simulink model "PositionControlNet"  (R2019b)
settings: Solver=ode3  StartTime=0.0  StopTime=100.0  FixedStep=Ts  RelTol=1e-3
values from neighbouring files (symbols this model uses):
  refx = 2.0    (= 2)    [RunPositionControl_b.m]    (also in RunPositionControl_d.m; RunPositionControl_e.m = 10 * rand - 5; RunPositionControl_i.m = 10 * rand - 5)
  refy = 2.0    (= 2)    [RunPositionControl_b.m]    (also in RunPositionControl_d.m; RunPositionControl_e.m = 10 * rand - 5; RunPositionControl_i.m = 10 * rand - 5)
undefined symbols (not defined in the file or in its folder): DiscIntNeverNeededParam
libraries: neural x56, simulink x1
(part 2 of 2)

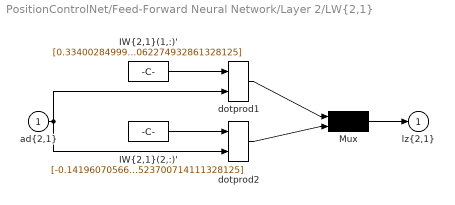
== system PositionControlNet/Feed-Forward Neural Network/Layer 2/LW{2,1} ==
  "ad{2,1}" : Inport  PortDimensions=50  SampleTime=0.1
      mask Display: e = 0.06;c1 = [120 230 180]/255;c2 = ([120 230 180]+0)/(256+128);c3 = ([120 230 180]+128)/(256+128);patch([0 1 1 0],[0 0 1 1],c1);patch([0 1 1 1-e 1-e 0+e],[0 0 1 1-e 0+e 0+e],c2);patch([0 0 1 1-e 0+e 0+e],[0 1 1 1-e 1-e 0+e],c3);plot([0 1 1 0 0],[0 0 1 1 0]);
  "IW{2,1}(1,:)'" : Constant  Value=[0.334002849994705253156013213811093010008335113525390625;-0.5040820987454741608502217786735855042934417724609375;-0.91935122834619387166554815848940052092075347900390625;0.32639735666295488503152455450617708265781402587890625;-0.187840693667216063200697817592299543321132659912109375;-0.11460469237998084646168450717595987953245639801025390625;0.717609320213467238858129348955117166042327880859375;1.3523732656893934223063524768804199993610382080078125;0.179703748271600349806220719983684830367565155029296875;-0.87500417966937893421430771923041902482509613037109375;-0.25199618840757465054736030651838518679141998291015625;-0.1195075191355988997177206556443707086145877838134765625;0.0728694591968338800658244736041524447500705718994140625;0.00809319958874362734013718778669499442912638187408447265625;-0.333437385428566102074654509124229662120342254638671875;0.0994025146375227264261553727919817902147769927978515625;-0.41078606437725884159561928754555992782115936279296875;0.60772390003159160176693376342882402241230010986328125;-0.50564194028696107796605474504758603870868682861328125;0.058621075153028744109118264304925105534493923187255859375;0.0248756429867585289461562325641352799721062183380126953125;-0.71916004594758631274231674979091621935367584228515625;-1.252886988501913823057520858128555119037628173828125;-0.1880074118303163566157110153653775341808795928955078125;0.1769309421471805532366516899855923838913440704345703125;0.47920092495693966672121177907683886587619781494140625;0.469176086459065333489348859075107611715793609619140625;0.377404235098586282592947327430010773241519927978515625;-0.406199561893793192890456111854291521012783050537109375;0.251041830696620227314497242332436144351959228515625;0.63316865040098979644511700826114974915981292724609375;-0.041829399940195056972758180791061022318899631500244140625;0.07987491955746865712750803822927991859614849090576171875;0.01011828325154251646822434196337781031616032123565673828125;0.0138200191255173875093387181323123513720929622650146484375;0.053368350017781542027339725109413848258554935455322265625;-0.62375837716052540127265046976390294730663299560546875;-0.045674105604766306043540424752791295759379863739013671875;-0.03509042242425212954071156445934320800006389617919921875;0.10806119620553211735369814050500281155109405517578125;-0.1630870104185702385013456705564749427139759063720703125;-0.11223416664183298585566461724738474003970623016357421875;-0.03950550369853102206096906456878059543669223785400390625;0.045018325314339573128830096493402379564940929412841796875;0.361073442667731503430417205890989862382411956787109375;-0.432799903513595152215742700718692503869533538818359375;0.984287018175489247795439951005391776561737060546875;0.125820475234998507829686786863021552562713623046875;-0.1203917071761672896723638359617325477302074432373046875;0.607004742466177305004748632200062274932861328125]
      mask Display: e = 0.06;c1 = [120 150 230]/255;c2 = ([120 150 230]+0)/383;c3 = ([120 150 230]+128)/383;patch([0 1 1 0],[0 0 1 1],c1);patch([0 1 1 1-e 1-e 0+e],[0 0 1 1-e 0+e 0+e],c2);patch([0 0 1 1-e 0+e 0+e],[0 1 1 1-e 1-e 0+e],c3);plot([0 1 1 0 0],[0 0 1 1 0]);disp('weights');
  "IW{2,1}(2,:)'" : Constant  Value=[-0.1419607056600145356117792516670306213200092315673828125;1.028827672248862068471453312668018043041229248046875;0.045383286118671088693599102725784177891910076141357421875;-0.218572716912245945675152825060649774968624114990234375;0.434083133810548360553838165287743322551250457763671875;0.50308140166235026935481755572254769504070281982421875;0.0201769956134996049368357518005723250098526477813720703125;0.04642214440832766186861846335887094028294086456298828125;-0.032438045155445953404704795275392825715243816375732421875;0.85025309020824313410713557459530420601367950439453125;-0.1201983909327605515304782102248282171785831451416015625;0.036994653062803813103887051738638547249138355255126953125;0.1300649198493276370580673528820625506341457366943359375;-0.344468723662421372200270752728101797401905059814453125;0.13513417310886577382689210935495793819427490234375;0.11122951518489221367502750581479631364345550537109375;-0.0789493036264423964087910690068383701145648956298828125;0.278793521052757231615260025137104094028472900390625;-0.08590393630611155295628833528098766691982746124267578125;0.0226878938136040701756268589406317914836108684539794921875;0.000776186346165941829823575748292796561145223677158355712890625;0.4489477159577852649618989744340069591999053955078125;0.1417734772799557896316713367923512123525142669677734375;-0.061852047013610460257648782089745509438216686248779296875;-0.2381090914265252267423278453861712478101253509521484375;0.274562097712392982895579507385264150798320770263671875;-0.0930798944562686025872011441606446169316768646240234375;-0.132101370043506471940730762071325443685054779052734375;0.0996268771357249616205109532529604621231555938720703125;0.261387848508712716810720166904502548277378082275390625;-0.0244297733572668984702858097080024890601634979248046875;-0.023142883803481929805290207013968029059469699859619140625;-0.0499752192089107649675128186572692357003688812255859375;-0.0179734345381963069032682511760867782868444919586181640625;0.014274641402173791904228750127003877423703670501708984375;0.129618086961626632902522260337718762457370758056640625;0.6746120176509069477077673582243733108043670654296875;-0.00854955465150222977677163527232551132328808307647705078125;-0.007409539415589941509232563277009830926544964313507080078125;-0.1792119123829565285888065773178823292255401611328125;0.0964519761765898764327431536003132350742816925048828125;0.0100209766125327025265701053058364777825772762298583984375;0.2555394827846504401946958751068450510501861572265625;0.0042921550021993680468224141577593400143086910247802734375;-0.43872622069355904361742659602896310389041900634765625;0.04703480228956517794625113992879050783812999725341796875;-0.9480305662744956674004015440004877746105194091796875;-0.050519411370737697664079490778021863661706447601318359375;0.017202658054994081349153844939792179502546787261962890625;-0.67035352331043640550234385955263860523700714111328125]
      mask Display: e = 0.06;c1 = [120 150 230]/255;c2 = ([120 150 230]+0)/383;c3 = ([120 150 230]+128)/383;patch([0 1 1 0],[0 0 1 1],c1);patch([0 1 1 1-e 1-e 0+e],[0 0 1 1-e 0+e 0+e],c2);patch([0 0 1 1-e 0+e 0+e],[0 1 1 1-e 1-e 0+e],c3);plot([0 1 1 0 0],[0 0 1 1 0]);disp('weights');
  Mux : Mux  Inputs=2
      mask Display: e = 0.06;c1 = [120 150 230]/255;c2 = ([120 150 230]+0)/383;c3 = ([120 150 230]+128)/383;patch([0 1 1 0],[0 0 1 1],c1);patch([0 1 1 1-e 1-e 0+e],[0 0 1 1-e 0+e 0+e],c2);patch([0 0 1 1-e 0+e 0+e],[0 1 1 1-e 1-e 0+e],c3);plot([0 1 1 0 0],[0 0 1 1 0]);disp('Mux');
  dotprod1 : neural/Weight Functions/dotprod
      settings: SourceProductName=Deep Learning Toolbox
  dotprod2 : neural/Weight Functions/dotprod
      settings: SourceProductName=Deep Learning Toolbox
  "lz{2,1}" : Outport
      mask Display: e = 0.06;c1 = [120 230 180]/255;c2 = ([120 230 180]+0)/(256+128);c3 = ([120 230 180]+128)/(256+128);patch([0 1 1 0],[0 0 1 1],c1);patch([0 1 1 1-e 1-e 0+e],[0 0 1 1-e 0+e 0+e],c2);patch([0 0 1 1-e 0+e 0+e],[0 1 1 1-e 1-e 0+e],c3);plot([0 1 1 0 0],[0 0 1 1 0]);
  wires:
  "IW{2,1}(1,:)'"/1 -> dotprod1/1
  "ad{2,1}"/1 -> dotprod1/2, dotprod2/2
  dotprod1/1 -> Mux/1
  "IW{2,1}(2,:)'"/1 -> dotprod2/1
  dotprod2/1 -> Mux/2
  Mux/1 -> "lz{2,1}"/1
